simulink model "LKARefMdl"  (R2020b)
settings: Solver=FixedStepAuto  StartTime=0.0  StopTime=simStopTime  FixedStep=1e-3  RelTol=1e-3
values from neighbouring files (symbols this model uses):
  gammann = 10000    [CreateNnMatrices.m]    (also in HvsNN.m = 0.01; MPC_Constrained_Control.m; MPC_NN.m = 1e+15)
  nc = n_c    (= 8)    [Model_Init_Bayes.m]
  np = n_p    (= 24)    [Model_Init_Bayes.m]
  numbConstr = 3*nc + 2*np    [CreateNnMatrices.m]    (also in HvsNN.m; MPC_Constrained_Control.m; MPC_NN.m)
  PredictionHorizon = 30    [helperLKASetUp.m]
  Ts = 0.1    [Model_Init_Bayes.m]    (also in helperLKASetUp.m)
undefined symbols (not defined in the file or in its folder): DiscIntNeverNeededParam, K
libraries: simulink x13, pid_lib x2
(part 1 of 2)
settings Model: Creator=The MathWorks, Inc.  LastModifiedBy=Stage
settings DataIOCC: SaveOutput=off  SaveTime=off  ReturnWorkspaceOutputs=off
settings OptimizationCC: DefaultParameterBehavior=Inlined  UseFloatMulNetSlope=on  DefaultUnderspecifiedDataType=single  UseSpecifiedMinMax=on  InlineInvariantSignals=on  EnhancedBackFolding=on  StrengthReduction=on  PassReuseOutputArgsAs=Individual arguments  ZeroExternalMemoryAtStartup=off  ZeroInternalMemoryAtStartup=off  NoFixptDivByZeroProtection=on  EfficientFloat2IntCast=on  OptimizeBlockOrder=speed  DifferentSizesBufferReuse=on  EfficientTunableParamExpr=on
settings DebuggingCC: ParameterPrecisionLossMsg=none  ParameterTunabilityLossMsg=error  ArithmeticOperatorsInVariantConditions=warning
settings HardwareCC: ProdLongLongMode=on
settings ModelReferenceCC: ModelReferenceNumInstancesAllowed=Single
settings SFSimCC: SimUseLocalCustomCode=off  MATLABDynamicMemAlloc=off  CustomCodeUndefinedFunction=UseInterfaceOnly  SimTargetLang=C++
settings RTWCC: Description=Embedded Coder  SystemTargetFile=ert.tlc  TemplateMakefile=ert_default_tmf  GenerateReport=on  RTWUseLocalCustomCode=off  BuildConfiguration=Faster Runs  IncludeHyperlinkInReport=on  LaunchReport=on  TargetLang=C++  GenerateTraceInfo=on  GenerateTraceReport=on  GenerateTraceReportSl=on  GenerateTraceReportSf=on  GenerateTraceReportEml=on
settings CodeAppCC: ForceParamTrailComments=on  IgnoreCustomStorageClasses=off  OperatorAnnotations=on  SimulinkDataObjDesc=on  SFDataObjDesc=on  InsertBlockDesc=on
settings ERTTargetCC: TargetLangStandard=C++03 (ISO)  GenerateSampleERTMain=on  CombineSignalStateStructs=on  SuppressErrorStatus=on  CodeInterfacePackaging=C++ class  InlinedParameterPlacement=NonHierarchical  RootIOFormat=Structure reference  ERTCustomFileTemplate=example_file_process.tlc

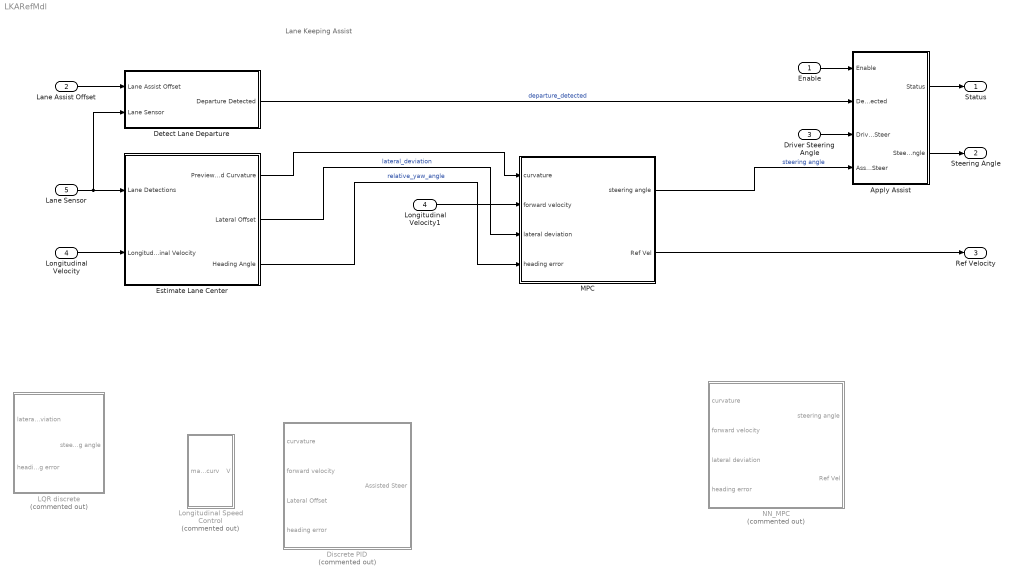
== system LKARefMdl ==
  note: Lane Keeping Assist
  Enable : Inport  OutDataTypeStr=boolean
  Lane Assist Offset : Inport  Port=2  OutDataTypeStr=single  Unit=m  SampleTime=Ts
  Driver Steering Angle : Inport  Port=3  Unit=rad
  Longitudinal Velocity : Inport  Port=4  OutDataTypeStr=single  Unit=m/s  SampleTime=Ts
  Lane Sensor : Inport  Port=5  OutDataTypeStr=Bus: LaneSensor  PortDimensions=[1 1]  SampleTime=Ts  BusOutputAsStruct=on
  Apply Assist : Subsystem
  Detect Lane Departure : Subsystem
  Discrete PID : Subsystem  Commented=on
  Estimate Lane Center : Subsystem  VariantControl=v2
  "LQR discrete " : Subsystem  Commented=on
  Longitudinal Speed Control : Subsystem  Commented=on
  Longitudinal Velocity1 : InportShadow  Port=4  OutDataTypeStr=single  Unit=m/s  SampleTime=Ts
  MPC : Subsystem
  NN_MPC : Subsystem  Commented=on
  Status : Outport  PortDimensions=1  VectorParamsAs1DForOutWhenUnconnected=off
  Steering Angle : Outport  Port=2  PortDimensions=1  VectorParamsAs1DForOutWhenUnconnected=off
  Ref Velocity : Outport  Port=3  PortDimensions=1  VectorParamsAs1DForOutWhenUnconnected=off
  wires:
  Estimate Lane Center/1(Previewed Curvature) -> MPC/1(curvature)
  Lane Assist Offset/1 -> Detect Lane Departure/1(Lane Assist Offset)
  Driver Steering Angle/1 -> Apply Assist/3(Driver Steer)
  Enable/1 -> Apply Assist/1(Enable)
  Apply Assist/1(Status) -> Status/1
  Apply Assist/2(Steering Angle) -> Steering Angle/1
  Detect Lane Departure/1(Departure Detected) -> Apply Assist/2(Departure Detected)  "departure_detected"
  Longitudinal Velocity/1 -> Estimate Lane Center/2(Longitudinal Velocity)
  Lane Sensor/1 -> Detect Lane Departure/2(Lane Sensor), Estimate Lane Center/1(Lane Detections)
  Estimate Lane Center/3(Heading Angle) -> MPC/4(heading error)  "relative_yaw_angle"
  Longitudinal Velocity1/1 -> MPC/2(forward velocity)
  MPC/2(Ref Vel) -> Ref Velocity/1
  MPC/1(steering angle) -> Apply Assist/4(Assisted Steer)  "steering angle"
  Estimate Lane Center/2(Lateral Offset) -> MPC/3(lateral deviation)  "lateral_deviation"

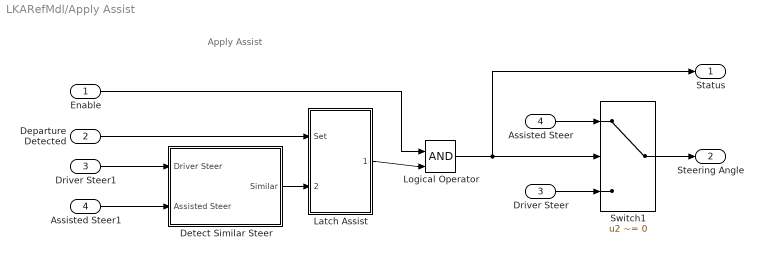
== system LKARefMdl/Apply Assist ==
  note: Apply Assist
  Enable : Inport
  Departure Detected : Inport  Port=2
  Driver Steer : Inport  Port=3
  Assisted Steer : Inport  Port=4
  Assisted Steer1 : InportShadow  Port=4
  "Detect Similar Steer " : Subsystem
  Driver Steer1 : InportShadow  Port=3
  Latch Assist : Subsystem
  Logical Operator : Logic  IconShape=distinctive  AllPortsSameDT=off  OutDataTypeStr=boolean
  Switch1 : Switch  Criteria=u2 ~= 0  Threshold=2
  Status : Outport  VectorParamsAs1DForOutWhenUnconnected=off
  Steering Angle : Outport  Port=2  Unit=rad  VectorParamsAs1DForOutWhenUnconnected=off
  wires:
  Assisted Steer/1 -> Switch1/1
  Driver Steer/1 -> Switch1/3
  Switch1/1 -> Steering Angle/1
  Enable/1 -> Logical Operator/1
  Logical Operator/1 -> Status/1, Switch1/2
  Driver Steer1/1 -> "Detect Similar Steer "/1(Driver Steer)
  Assisted Steer1/1 -> "Detect Similar Steer "/2(Assisted Steer)
  Departure Detected/1 -> Latch Assist/1(Set)
  "Detect Similar Steer "/1(Similar) -> Latch Assist/2(Reset)
  Latch Assist/1(Assist) -> Logical Operator/2

== system LKARefMdl/Detect Lane Departure ==
  note: Detect Lane Departure
  Lane Assist Offset : Inport
  In Bus Element : Inport  Port=2  PortName=Lane Sensor  Element=Left.LateralOffset
  In Bus Element1 : Inport  Port=2  PortName=Lane Sensor  Element=Right.LateralOffset
  Gain : Gain  Gain=-1
  Lane Assist Offset1 : InportShadow
  Logical Operator : Logic  Operator=OR  IconShape=distinctive  AllPortsSameDT=off  OutDataTypeStr=boolean
  Relational Operator : RelationalOperator  Operator=<=  OutDataTypeStr=boolean  RndMeth=Simplest
  Relational Operator1 : RelationalOperator  OutDataTypeStr=boolean  RndMeth=Simplest
  Departure Detected : Outport  VectorParamsAs1DForOutWhenUnconnected=off
  wires:
  Lane Assist Offset/1 -> Relational Operator/2  "left_assist_offset"
  In Bus Element/1 -> Relational Operator/1  "left_lateral_offset"
  Lane Assist Offset1/1 -> Gain/1  "left_assist_offset"
  In Bus Element1/1 -> Relational Operator1/1  "right_lateral_offset"
  Gain/1 -> Relational Operator1/2  "right_assist_offset"
  Relational Operator/1 -> Logical Operator/1
  Relational Operator1/1 -> Logical Operator/2
  Logical Operator/1 -> Departure Detected/1

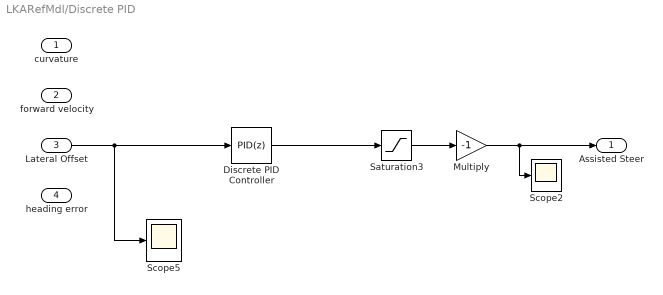
== system LKARefMdl/Discrete PID ==
  curvature : Inport
  forward velocity : Inport  Port=2
  Lateral Offset : Inport  Port=3
  heading error : Inport  Port=4
  Discrete PID Controller : pid_lib/PID Controller  Controller=PID  Form=Parallel  TimeDomain=Discrete-time  UseExternalTs=off  SampleTime=-1  IntegratorMethod=Forward Euler  FilterMethod=Forward Euler  ControllerParametersSource=internal  P=.5  I=.1  D=1  UseFilter=off  N=100  TunerSelectOption=Transfer Function Based (PID Tuner App)  InitialConditionSource=internal  InitialConditionForIntegrator=0  InitialConditionForFilter=0  DifferentiatorICPrevScaledInput=0  ExternalReset=none  TrackingMode=off  Kt=1  LimitOutput=off  SatLimitsSource=internal  UpperSaturationLimit=inf  LowerSaturationLimit=-inf  LinearizeAsGain=off  AntiWindupMode=none  Kb=1  POutMin=[]  POutMax=[]  IOutMin=[]  IOutMax=[]  DOutMin=[]  DOutMax=[]  NOutMin=[]  NOutMax=[]  SumOutMin=[]  SumOutMax=[]  SaturationOutMin=[]  SaturationOutMax=[]  PParamMin=[]  PParamMax=[]  IParamMin=[]  IParamMax=[]  DParamMin=[]  DParamMax=[]  NParamMin=[]  NParamMax=[]  KbParamMin=[]  KbParamMax=[]  KtParamMin=[]  KtParamMax=[]  KbOutMin=[]  KbOutMax=[]  KtOutMin=[]  KtOutMax=[]  IntegratorOutMin=[]  IntegratorOutMax=[]  FilterOutMin=[]  FilterOutMax=[]  SumI1OutMin=[]  SumI1OutMax=[]  SumI2OutMin=[]  SumI2OutMax=[]  SumI3OutMin=[]  SumI3OutMax=[]  SumI4OutMin=[]  SumI4OutMax=[]  SumDOutMin=[]  SumDOutMax=[]  DifferentiatorOutMin=[]  DifferentiatorOutMax=[]  FilterDiffOutCoefMin=[]  FilterDiffOutCoefMax=[]  ReciprocalOutMin=[]  ReciprocalOutMax=[]  SumDenOutMin=[]  SumDenOutMax=[]  SumNumOutMin=[]  SumNumOutMax=[]  DivideOutMin=[]  DivideOutMax=[]  UdiffTsProdOutMin=[]  UdiffTsProdOutMax=[]  NTsProdOutMin=[]  NTsProdOutMax=[]  UintegralTsProdOutMin=[]  UintegralTsProdOutMax=[]  UngainTsProdOutMin=[]  UngainTsProdOutMax=[]  IntegratorContinuousStateAttributes=''  IntegratorStateMustResolveToSignalObject=off  IntegratorRTWStateStorageClass=Auto  FilterContinuousStateAttributes=''  FilterStateMustResolveToSignalObject=off  FilterRTWStateStorageClass=Auto  ParallelPVariant=InternalParameters  IdealPVariant=Disabled  IVariant=InternalParameters  DVariant=InternalParameters  IntegratorVariant=Discrete  SatVariant=Disabled  AWVariant=Passthrough  PCopyVariant=Disabled  TRVariant=Disabled  FdbkBlocksVariant=Forward  IdealPFdbkVariant=Disabled  SatFdbkVariant=Disabled  DerivativeFilterVariant=Differentiator  NVariant=Passthrough  NCopyVariant=Disabled_SignalSpec  FilterICVariant=InternalICsDifferentiator  IntegratorICVariant=InternalICs  ExternalResetVariant=Disabled  TRSumVariant=Passthrough  SumFdbkVariant=Disabled  SumVariant=Sum_PID  TsampFilterVariant=InternalTs  TsampNgainVariant=Passthrough  TsampIntegralVariant=Passthrough  ExternalSaturationOutDataTypeStr=Inherit: Same as second input
  Multiply : Gain  Gain=-1
  Saturation3 : Saturate
  Scope2 : Scope
  Scope5 : Scope
  Assisted Steer : Outport
  wires:
  Lateral Offset/1 -> Discrete PID Controller/1, Scope5/1
  Discrete PID Controller/1 -> Saturation3/1
  Saturation3/1 -> Multiply/1
  Multiply/1 -> Scope2/1, Assisted Steer/1

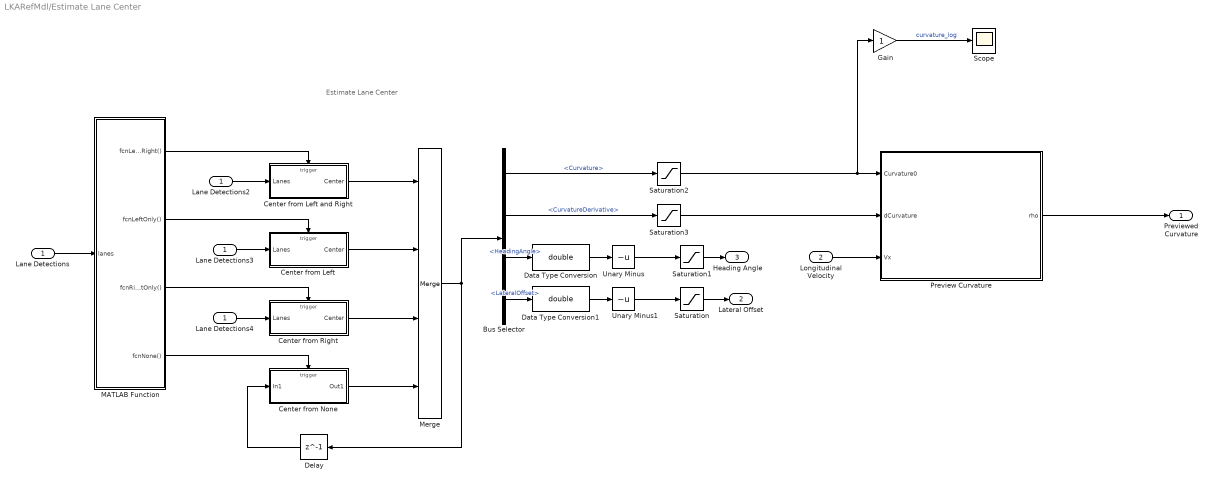
== system LKARefMdl/Estimate Lane Center ==
  note: Estimate Lane Center
  Lane Detections : Inport
  Longitudinal Velocity : Inport  Port=2  OutDataTypeStr=single
  Bus Selector : BusSelector  OutputSignals=Curvature,CurvatureDerivative,HeadingAngle,LateralOffset
  Center from Left : Subsystem  TreatAsAtomicUnit=on
  Center from Left and Right : Subsystem  TreatAsAtomicUnit=on
  Center from None : Subsystem  TreatAsAtomicUnit=on
  Center from Right : Subsystem  TreatAsAtomicUnit=on
  Data Type Conversion : DataTypeConversion  OutDataTypeStr=double
  Data Type Conversion1 : DataTypeConversion  OutDataTypeStr=double
  Delay : Delay  DelayLength=1
  Gain : Gain
  Lane Detections2 : InportShadow
  Lane Detections3 : InportShadow
  Lane Detections4 : InportShadow
  MATLAB Function : MATLAB Function  TreatAsAtomicUnit=on
  Merge : Merge  Inputs=4
  Preview Curvature : MATLAB Function  TreatAsAtomicUnit=on  SystemSampleTime=Ts
  Saturation : Saturate
  Saturation1 : Saturate  UpperLimit=0.6  LowerLimit=-0.6
  Saturation2 : Saturate  UpperLimit=0.15  LowerLimit=-0.15
  Saturation3 : Saturate  UpperLimit=0.06  LowerLimit=-0.06
  Scope : Scope
  Unary Minus : UnaryMinus
  Unary Minus1 : UnaryMinus
  Previewed Curvature : Outport  VectorParamsAs1DForOutWhenUnconnected=off
  Lateral Offset : Outport  Port=2  VectorParamsAs1DForOutWhenUnconnected=off
  Heading Angle : Outport  Port=3  VectorParamsAs1DForOutWhenUnconnected=off
  wires:
  Bus Selector/3 -> Data Type Conversion/1  "<HeadingAngle>"
  Bus Selector/4 -> Data Type Conversion1/1  "<LateralOffset>"
  Unary Minus1/1 -> Saturation/1
  Bus Selector/1 -> Saturation2/1  "<Curvature>"
  Bus Selector/2 -> Saturation3/1  "<CurvatureDerivative>"
  Longitudinal Velocity/1 -> Preview Curvature/3(Vx)
  Unary Minus/1 -> Saturation1/1
  Saturation/1 -> Lateral Offset/1
  Saturation1/1 -> Heading Angle/1
  Saturation3/1 -> Preview Curvature/2(dCurvature)
  Merge/1 -> Delay/1, Bus Selector/1
  Center from Left/1(Center) -> Merge/2
  MATLAB Function/4(fcnNone()) -> Center from None/Trigger
  MATLAB Function/3(fcnRightOnly()) -> Center from Right/Trigger
  Lane Detections2/1 -> Center from Left and Right/1(Lanes)
  Lane Detections/1 -> MATLAB Function/1(lanes)
  Center from Left and Right/1(Center) -> Merge/1
  Delay/1 -> Center from None/1(In1)
  MATLAB Function/1(fcnLeftAndRight()) -> Center from Left and Right/Trigger
  Center from None/1(Out1) -> Merge/4
  MATLAB Function/2(fcnLeftOnly()) -> Center from Left/Trigger
  Lane Detections4/1 -> Center from Right/1(Lanes)
  Lane Detections3/1 -> Center from Left/1(Lanes)
  Center from Right/1(Center) -> Merge/3
  Data Type Conversion/1 -> Unary Minus/1
  Data Type Conversion1/1 -> Unary Minus1/1
  Preview Curvature/1(rho) -> Previewed Curvature/1
  Gain/1 -> Scope/1  "curvature_log"
  Saturation2/1 -> Gain/1, Preview Curvature/1(Curvature0)

== system LKARefMdl/LQR discrete  ==
  lateral deviation : Inport
  heading error : Inport  Port=2
  Discrete Derivative : simulink/Discrete/Discrete Derivative  gainval=1.0  ICPrevScaledInput=0.0  OutMin=[]  OutMax=[]  OutDataType=fixdt(1, 16)  OutScaling=2^-10  DoSatur=off
  Discrete Derivative1 : simulink/Discrete/Discrete Derivative  gainval=1.0  ICPrevScaledInput=0.012353340233836  OutMin=[]  OutMax=[]  OutDataType=fixdt(1, 16)  OutScaling=2^-10  DoSatur=off
  Multiply : Gain  Gain=-K  Multiplication=Matrix(K*u) (u vector)
  Mux : Mux
  Saturation : Saturate  UpperLimit=0.4  LowerLimit=-0.4
  steering angle : Outport
  wires:
  Multiply/1 -> Saturation/1
  Saturation/1 -> steering angle/1
  Discrete Derivative1/1 -> Mux/4
  Discrete Derivative/1 -> Mux/2
  Mux/1 -> Multiply/1
  lateral deviation/1 -> Discrete Derivative/1, Mux/1
  heading error/1 -> Mux/3, Discrete Derivative1/1

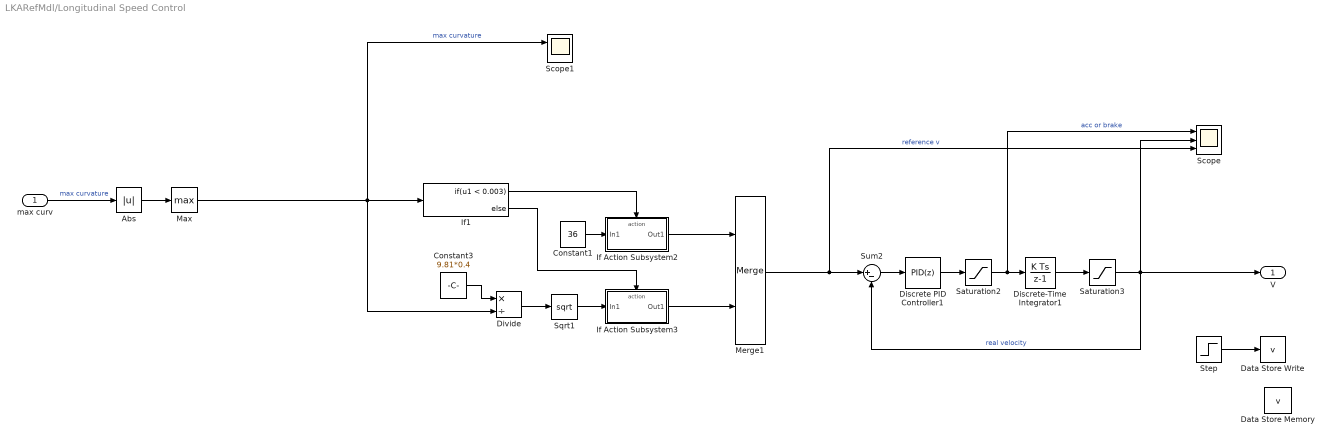
== system LKARefMdl/Longitudinal Speed Control ==
  max curv : Inport
  Abs : Abs
  Constant1 : Constant  Value=36
  Constant3 : Constant  Value=9.81*0.4
  Data Store Memory : DataStoreMemory  DataStoreName=v  ReadBeforeWriteMsg=warning  WriteAfterWriteMsg=warning  WriteAfterReadMsg=warning  ShowAdditionalParam=off  OutDataTypeStr=double
  Data Store Write : DataStoreWrite  DataStoreName=v  DataStoreElements=v
  Discrete PID Controller1 : pid_lib/PID Controller  Controller=PID  Form=Parallel  TimeDomain=Discrete-time  UseExternalTs=off  SampleTime=Ts  IntegratorMethod=Forward Euler  FilterMethod=Forward Euler  ControllerParametersSource=internal  P=7  I=0  D=0  UseFilter=on  N=100  TunerSelectOption=Transfer Function Based (PID Tuner App)  InitialConditionSource=internal  InitialConditionForIntegrator=0  InitialConditionForFilter=0  DifferentiatorICPrevScaledInput=0  ExternalReset=none  TrackingMode=off  Kt=1  LimitOutput=off  SatLimitsSource=internal  UpperSaturationLimit=inf  LowerSaturationLimit=-inf  LinearizeAsGain=off  AntiWindupMode=none  Kb=1  POutMin=[]  POutMax=[]  IOutMin=[]  IOutMax=[]  DOutMin=[]  DOutMax=[]  NOutMin=[]  NOutMax=[]  SumOutMin=[]  SumOutMax=[]  SaturationOutMin=[]  SaturationOutMax=[]  PParamMin=[]  PParamMax=[]  IParamMin=[]  IParamMax=[]  DParamMin=[]  DParamMax=[]  NParamMin=[]  NParamMax=[]  KbParamMin=[]  KbParamMax=[]  KtParamMin=[]  KtParamMax=[]  KbOutMin=[]  KbOutMax=[]  KtOutMin=[]  KtOutMax=[]  IntegratorOutMin=[]  IntegratorOutMax=[]  FilterOutMin=[]  FilterOutMax=[]  SumI1OutMin=[]  SumI1OutMax=[]  SumI2OutMin=[]  SumI2OutMax=[]  SumI3OutMin=[]  SumI3OutMax=[]  SumI4OutMin=[]  SumI4OutMax=[]  SumDOutMin=[]  SumDOutMax=[]  DifferentiatorOutMin=[]  DifferentiatorOutMax=[]  FilterDiffOutCoefMin=[]  FilterDiffOutCoefMax=[]  ReciprocalOutMin=[]  ReciprocalOutMax=[]  SumDenOutMin=[]  SumDenOutMax=[]  SumNumOutMin=[]  SumNumOutMax=[]  DivideOutMin=[]  DivideOutMax=[]  UdiffTsProdOutMin=[]  UdiffTsProdOutMax=[]  NTsProdOutMin=[]  NTsProdOutMax=[]  UintegralTsProdOutMin=[]  UintegralTsProdOutMax=[]  UngainTsProdOutMin=[]  UngainTsProdOutMax=[]  IntegratorContinuousStateAttributes=''  IntegratorStateMustResolveToSignalObject=off  IntegratorRTWStateStorageClass=Auto  FilterContinuousStateAttributes=''  FilterStateMustResolveToSignalObject=off  FilterRTWStateStorageClass=Auto  ParallelPVariant=InternalParameters  IdealPVariant=Disabled  IVariant=InternalParameters  DVariant=InternalParameters  IntegratorVariant=Discrete  SatVariant=Disabled  AWVariant=Passthrough  PCopyVariant=Disabled  TRVariant=Disabled  FdbkBlocksVariant=Forward  IdealPFdbkVariant=Disabled  SatFdbkVariant=Disabled  DerivativeFilterVariant=ForwardEulerFilter  NVariant=InternalParameters  NCopyVariant=Disabled  FilterICVariant=InternalICsFilter  IntegratorICVariant=InternalICs  ExternalResetVariant=Disabled  TRSumVariant=Passthrough  SumFdbkVariant=Disabled  SumVariant=Sum_PID  TsampFilterVariant=InternalTs  TsampNgainVariant=Passthrough  TsampIntegralVariant=Passthrough  ExternalSaturationOutDataTypeStr=Inherit: Same as second input
  Discrete-Time Integrator1 : DiscreteIntegrator  SampleTime=Ts  ICPrevOutput=DiscIntNeverNeededParam  ICPrevScaledInput=DiscIntNeverNeededParam
  Divide : Product  Inputs=*/
  If Action Subsystem2 : Subsystem  TreatAsAtomicUnit=on
  If Action Subsystem3 : Subsystem  TreatAsAtomicUnit=on
  If1 : If  IfExpression=u1 < 0.003
  Max : MinMax  Function=max
  Merge1 : Merge
  Saturation2 : Saturate  UpperLimit=0.5*9.81  LowerLimit=-0.5*9.81
  Saturation3 : Saturate  UpperLimit=36  LowerLimit=0
  Scope : Scope  NumInputPorts=3
  Scope1 : Scope  NumInputPorts=2
  Sqrt1 : Sqrt  SaturateOnIntegerOverflow=on
  Step : Step  Time=5  Before=2  After=7  SampleTime=0
  Sum2 : Sum  Inputs=|+-
  V : Outport
  wires:
  Saturation3/1 -> V/1, Sum2/2, Scope/2  "real velocity"
  Saturation2/1 -> Scope/1, Discrete-Time Integrator1/1  "acc or brake"
  Discrete-Time Integrator1/1 -> Saturation3/1
  Discrete PID Controller1/1 -> Saturation2/1
  Sum2/1 -> Discrete PID Controller1/1
  Merge1/1 -> Scope/3, Sum2/1  "reference v"
  If1/1 -> If Action Subsystem2/Action
  Constant3/1 -> Divide/1
  Max/1 -> Divide/2, Scope1/1, If1/1  "max curvature"
  Constant1/1 -> If Action Subsystem2/1(In1)
  If Action Subsystem2/1(Out1) -> Merge1/1
  Divide/1 -> Sqrt1/1
  Sqrt1/1 -> If Action Subsystem3/1(In1)
  If1/2 -> If Action Subsystem3/Action
  If Action Subsystem3/1(Out1) -> Merge1/2
  Step/1 -> Data Store Write/1
  Abs/1 -> Max/1
  max curv/1 -> Abs/1  "max curvature"

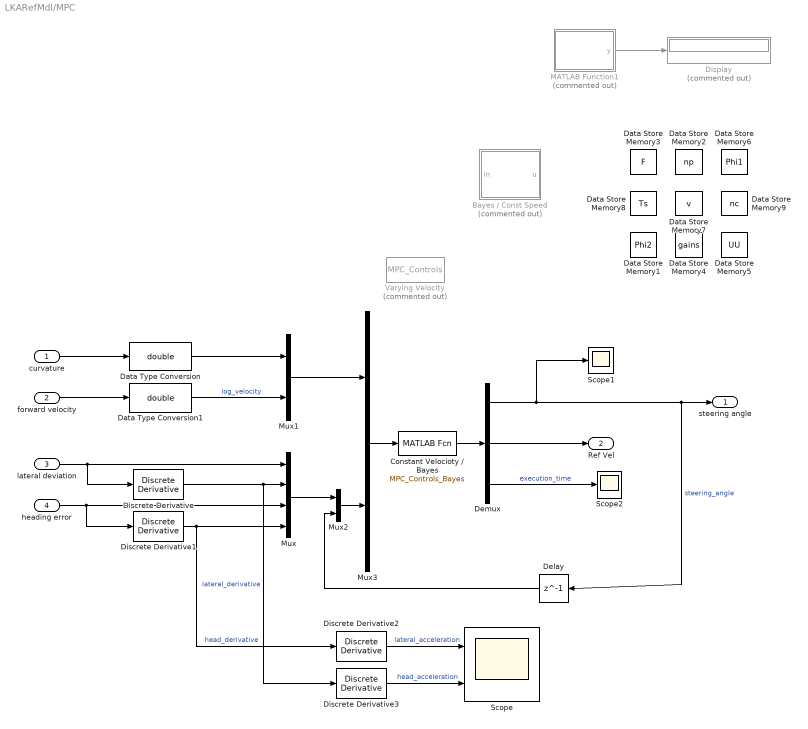
== system LKARefMdl/MPC ==
  curvature : Inport
  forward velocity : Inport  Port=2
  lateral deviation : Inport  Port=3
  heading error : Inport  Port=4
  Bayes / Const Speed : MATLAB Function  Commented=on  TreatAsAtomicUnit=on
  Constant Velocioty / Bayes : MATLABFcn  MATLABFcn=MPC_Controls_Bayes  OutputDimensions=3  OutputSignalType=real  Output1D=off
  Data Store Memory1 : DataStoreMemory  DataStoreName=Phi2  WriteAfterWriteMsg=warning  WriteAfterReadMsg=warning  InitialValue=Phi2  ShowAdditionalParam=off  OutDataTypeStr=double
  Data Store Memory2 : DataStoreMemory  DataStoreName=np  WriteAfterWriteMsg=warning  WriteAfterReadMsg=warning  InitialValue=np  ShowAdditionalParam=off  OutDataTypeStr=double
  Data Store Memory3 : DataStoreMemory  DataStoreName=F  WriteAfterWriteMsg=warning  WriteAfterReadMsg=warning  InitialValue=F  ShowAdditionalParam=off  OutDataTypeStr=double
  Data Store Memory4 : DataStoreMemory  DataStoreName=gains  WriteAfterWriteMsg=warning  WriteAfterReadMsg=warning  InitialValue=gains  ShowAdditionalParam=off  OutDataTypeStr=double
  Data Store Memory5 : DataStoreMemory  DataStoreName=UU  WriteAfterWriteMsg=warning  WriteAfterReadMsg=warning  InitialValue=UU  ShowAdditionalParam=off  OutDataTypeStr=double
  Data Store Memory6 : DataStoreMemory  DataStoreName=Phi1  WriteAfterWriteMsg=warning  WriteAfterReadMsg=warning  InitialValue=Phi2  ShowAdditionalParam=off  OutDataTypeStr=double
  Data Store Memory7 : DataStoreMemory  DataStoreName=v  WriteAfterWriteMsg=warning  WriteAfterReadMsg=warning  InitialValue=v  ShowAdditionalParam=off  OutDataTypeStr=double
  Data Store Memory8 : DataStoreMemory  DataStoreName=Ts  WriteAfterWriteMsg=warning  WriteAfterReadMsg=warning  InitialValue=Ts  ShowAdditionalParam=off  OutDataTypeStr=double
  Data Store Memory9 : DataStoreMemory  DataStoreName=nc  WriteAfterWriteMsg=warning  WriteAfterReadMsg=warning  InitialValue=nc  ShowAdditionalParam=off  OutDataTypeStr=double
  Data Type Conversion : DataTypeConversion  OutDataTypeStr=double
  Data Type Conversion1 : DataTypeConversion  OutDataTypeStr=double
  Delay : Delay  DelayLength=1  InitialCondition=0
  Demux : Demux  Outputs=3
  Discrete Derivative : simulink/Discrete/Discrete Derivative  gainval=1.0  ICPrevScaledInput=10  OutMin=[]  OutMax=[]  OutDataType=fixdt(1, 16)  OutScaling=2^-10  DoSatur=off
  Discrete Derivative1 : simulink/Discrete/Discrete Derivative  gainval=1.0  ICPrevScaledInput=0.0  OutMin=[]  OutMax=[]  OutDataType=fixdt(1, 16)  OutScaling=2^-10  DoSatur=off
  Discrete Derivative2 : simulink/Discrete/Discrete Derivative  gainval=1.0  ICPrevScaledInput=10  OutMin=[]  OutMax=[]  OutDataType=fixdt(1, 16)  OutScaling=2^-10  DoSatur=off
  Discrete Derivative3 : simulink/Discrete/Discrete Derivative  gainval=1.0  ICPrevScaledInput=0.0  OutMin=[]  OutMax=[]  OutDataType=fixdt(1, 16)  OutScaling=2^-10  DoSatur=off
  Display : Display  Commented=on
  MATLAB Function1 : MATLAB Function  Commented=on  TreatAsAtomicUnit=on
  Mux : Mux
  Mux1 : Mux  Inputs=2
  Mux2 : Mux  Inputs=2
  Mux3 : Mux  Inputs=2
  Scope : Scope  NumInputPorts=2
  Scope1 : Scope
  Scope2 : Scope
  Varying Velocity : MATLABFcn  Commented=on  MATLABFcn=MPC_Controls  OutputDimensions=2  OutputSignalType=real  Output1D=off
  steering angle : Outport
  Ref Vel : Outport  Port=2
  wires:
  Constant Velocioty / Bayes/1 -> Demux/1
  Mux3/1 -> Constant Velocioty / Bayes/1
  Discrete Derivative2/1 -> Scope/1  "lateral_acceleration"
  Discrete Derivative3/1 -> Scope/2  "head_acceleration"
  Delay/1 -> Mux2/2
  Demux/2 -> Ref Vel/1
  Data Type Conversion1/1 -> Mux1/2  "log_velocity"
  MATLAB Function1/1(y) -> Display/1
  Mux1/1 -> Mux3/1
  Mux2/1 -> Mux3/2
  Mux/1 -> Mux2/1
  Data Type Conversion/1 -> Mux1/1
  forward velocity/1 -> Data Type Conversion1/1
  Demux/1 -> Delay/1, steering angle/1, Scope1/1  "steering_angle"
  Discrete Derivative/1 -> Discrete Derivative3/1, Mux/2  "lateral_derivative"
  Discrete Derivative1/1 -> Mux/4, Discrete Derivative2/1  "head_derivative"
  heading error/1 -> Mux/3, Discrete Derivative1/1
  lateral deviation/1 -> Discrete Derivative/1, Mux/1
  curvature/1 -> Data Type Conversion/1
  Demux/3 -> Scope2/1  "execution_time"

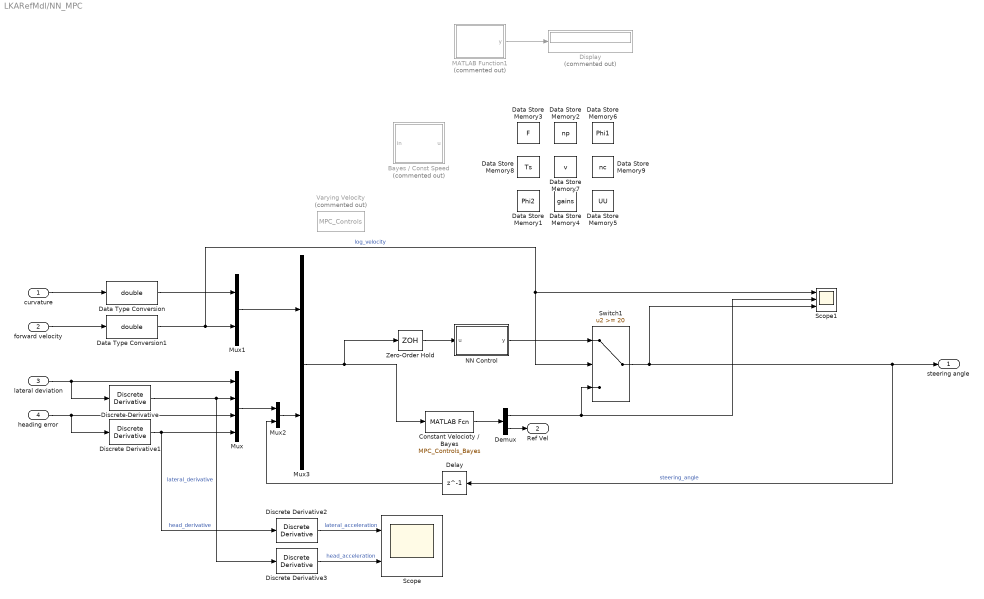
== system LKARefMdl/NN_MPC ==
  curvature : Inport
  forward velocity : Inport  Port=2
  lateral deviation : Inport  Port=3
  heading error : Inport  Port=4
  Bayes / Const Speed : MATLAB Function  Commented=on  TreatAsAtomicUnit=on
  Constant Velocioty / Bayes : MATLABFcn  MATLABFcn=MPC_Controls_Bayes  OutputDimensions=2  OutputSignalType=real  Output1D=off
  Data Store Memory1 : DataStoreMemory  DataStoreName=Phi2  WriteAfterWriteMsg=warning  WriteAfterReadMsg=warning  InitialValue=Phi2  ShowAdditionalParam=off  OutDataTypeStr=double
  Data Store Memory2 : DataStoreMemory  DataStoreName=np  WriteAfterWriteMsg=warning  WriteAfterReadMsg=warning  InitialValue=np  ShowAdditionalParam=off  OutDataTypeStr=double
  Data Store Memory3 : DataStoreMemory  DataStoreName=F  WriteAfterWriteMsg=warning  WriteAfterReadMsg=warning  InitialValue=F  ShowAdditionalParam=off  OutDataTypeStr=double
  Data Store Memory4 : DataStoreMemory  DataStoreName=gains  WriteAfterWriteMsg=warning  WriteAfterReadMsg=warning  InitialValue=gains  ShowAdditionalParam=off  OutDataTypeStr=double
  Data Store Memory5 : DataStoreMemory  DataStoreName=UU  WriteAfterWriteMsg=warning  WriteAfterReadMsg=warning  InitialValue=UU  ShowAdditionalParam=off  OutDataTypeStr=double
  Data Store Memory6 : DataStoreMemory  DataStoreName=Phi1  WriteAfterWriteMsg=warning  WriteAfterReadMsg=warning  InitialValue=Phi1  ShowAdditionalParam=off  OutDataTypeStr=double
  Data Store Memory7 : DataStoreMemory  DataStoreName=v  WriteAfterWriteMsg=warning  WriteAfterReadMsg=warning  InitialValue=v  ShowAdditionalParam=off  OutDataTypeStr=double
  Data Store Memory8 : DataStoreMemory  DataStoreName=Ts  WriteAfterWriteMsg=warning  WriteAfterReadMsg=warning  InitialValue=Ts  ShowAdditionalParam=off  OutDataTypeStr=double
  Data Store Memory9 : DataStoreMemory  DataStoreName=nc  WriteAfterWriteMsg=warning  WriteAfterReadMsg=warning  InitialValue=nc  ShowAdditionalParam=off  OutDataTypeStr=double
  Data Type Conversion : DataTypeConversion  OutDataTypeStr=double
  Data Type Conversion1 : DataTypeConversion  OutDataTypeStr=double
  Delay : Delay  DelayLength=1  InitialCondition=0  SampleTime=Ts
  Demux : Demux  Outputs=2
  Discrete Derivative : simulink/Discrete/Discrete Derivative  gainval=1.0  ICPrevScaledInput=10  OutMin=[]  OutMax=[]  OutDataType=fixdt(1, 16)  OutScaling=2^-10  DoSatur=off
  Discrete Derivative1 : simulink/Discrete/Discrete Derivative  gainval=1.0  ICPrevScaledInput=0.0  OutMin=[]  OutMax=[]  OutDataType=fixdt(1, 16)  OutScaling=2^-10  DoSatur=off
  Discrete Derivative2 : simulink/Discrete/Discrete Derivative  gainval=1.0  ICPrevScaledInput=10  OutMin=[]  OutMax=[]  OutDataType=fixdt(1, 16)  OutScaling=2^-10  DoSatur=off
  Discrete Derivative3 : simulink/Discrete/Discrete Derivative  gainval=1.0  ICPrevScaledInput=0.0  OutMin=[]  OutMax=[]  OutDataType=fixdt(1, 16)  OutScaling=2^-10  DoSatur=off
  Display : Display  Commented=on
  MATLAB Function1 : MATLAB Function  Commented=on  TreatAsAtomicUnit=on
  Mux : Mux
  Mux1 : Mux  Inputs=2
  Mux2 : Mux  Inputs=2
  Mux3 : Mux  Inputs=2
  NN Control : Subsystem  TreatAsAtomicUnit=on
  Scope : Scope  NumInputPorts=2
  Scope1 : Scope  NumInputPorts=3
  Switch1 : Switch  Threshold=20
  Varying Velocity : MATLABFcn  Commented=on  MATLABFcn=MPC_Controls  OutputDimensions=2  OutputSignalType=real  Output1D=off
  Zero-Order Hold : ZeroOrderHold  SampleTime=0.00000001
  steering angle : Outport
  Ref Vel : Outport  Port=2
  wires:
  curvature/1 -> Data Type Conversion/1
  lateral deviation/1 -> Mux/1, Discrete Derivative/1
  heading error/1 -> Discrete Derivative1/1, Mux/3
  Discrete Derivative1/1 -> Discrete Derivative2/1, Mux/4  "head_derivative"
  Discrete Derivative/1 -> Mux/2, Discrete Derivative3/1  "lateral_derivative"
  Switch1/1 -> Scope1/3, steering angle/1, Delay/1  "steering_angle"
  forward velocity/1 -> Data Type Conversion1/1
  Data Type Conversion/1 -> Mux1/1
  Mux/1 -> Mux2/1
  Mux2/1 -> Mux3/2
  Mux1/1 -> Mux3/1
  MATLAB Function1/1(y) -> Display/1
  Data Type Conversion1/1 -> Scope1/1, Switch1/2, Mux1/2  "log_velocity"
  Delay/1 -> Mux2/2
  Discrete Derivative3/1 -> Scope/2  "head_acceleration"
  Discrete Derivative2/1 -> Scope/1  "lateral_acceleration"
  Mux3/1 -> Constant Velocioty / Bayes/1, Zero-Order Hold/1
  Demux/2 -> Ref Vel/1
  Constant Velocioty / Bayes/1 -> Demux/1
  Demux/1 -> Scope1/2, Switch1/3
  NN Control/1(y) -> Switch1/1
  Zero-Order Hold/1 -> NN Control/1(u)

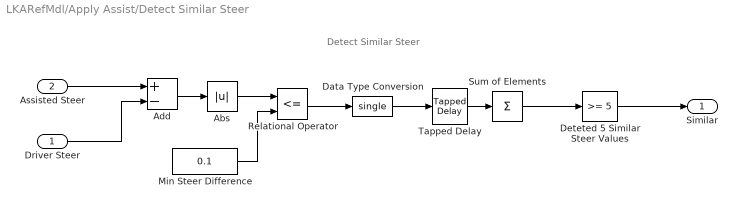
== system LKARefMdl/Apply Assist/Detect Similar Steer  ==
  note: Detect Similar Steer
  Driver Steer : Inport
  Assisted Steer : Inport  Port=2
  Abs : Abs
  Add : Sum  Inputs=+-
  Data Type Conversion : DataTypeConversion  OutDataTypeStr=single
  Deteted 5 Similar Steer Values : simulink/Logic and Bit Operations/Compare To Constant  relop=>=  const=5  OutDataTypeStr=boolean
  Min Steer Difference : Constant  Value=0.1
  Relational Operator : RelationalOperator  Operator=<=  OutDataTypeStr=boolean  RndMeth=Simplest
  Sum of Elements : Sum  Inputs=+
  Tapped Delay : simulink/Discrete/Tapped Delay  vinit=0.0  samptime=-1  NumDelays=5  DelayOrder=Oldest  includeCurrent=off
  Similar : Outport  VectorParamsAs1DForOutWhenUnconnected=off
  wires:
  Assisted Steer/1 -> Add/1
  Driver Steer/1 -> Add/2
  Add/1 -> Abs/1
  Relational Operator/1 -> Data Type Conversion/1
  Abs/1 -> Relational Operator/1
  Deteted 5 Similar Steer Values/1 -> Similar/1
  Min Steer Difference/1 -> Relational Operator/2
  Data Type Conversion/1 -> Tapped Delay/1
  Tapped Delay/1 -> Sum of Elements/1
  Sum of Elements/1 -> Deteted 5 Similar Steer Values/1

== system LKARefMdl/Apply Assist/Latch Assist ==
  note: Latch Assist
  Set : Inport
  Reset : Inport  Port=2
  Delay : Delay  DelayLength=1
  Logical Operator1 : Logic  Operator=OR  IconShape=distinctive  AllPortsSameDT=off  OutDataTypeStr=boolean
  Logical Operator2 : Logic  IconShape=distinctive  AllPortsSameDT=off  OutDataTypeStr=boolean
  Logical Operator3 : Logic  Operator=NOT  IconShape=distinctive  AllPortsSameDT=off  OutDataTypeStr=boolean
  Assist : Outport  VectorParamsAs1DForOutWhenUnconnected=off
  wires:
  Logical Operator1/1 -> Assist/1, Delay/1  "latch_assist"
  Delay/1 -> Logical Operator2/2
  Reset/1 -> Logical Operator3/1
  Logical Operator2/1 -> Logical Operator1/2  "unlatch_assist"
  Set/1 -> Logical Operator1/1
  Logical Operator3/1 -> Logical Operator2/1

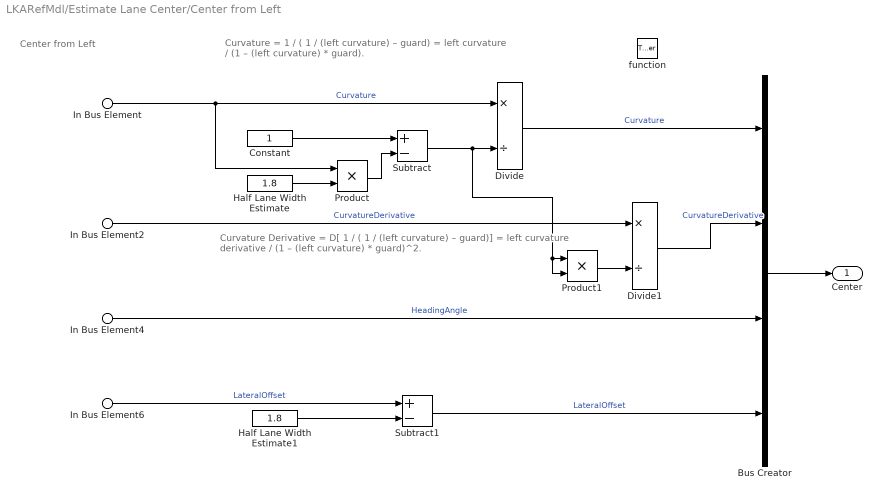
== system LKARefMdl/Estimate Lane Center/Center from Left ==
  note: Curvature
      | = 1 / ( 1 / (left curvature) – guard)
      | = left curvature / (1 – (left curvature) * guard).
  note: Center from Left
  note: Curvature Derivative
      | = D[ 1 / ( 1 / (left curvature) – guard)]
      | = left curvature derivative / (1 – (left curvature) * guard)^2.
  In Bus Element : Inport  PortName=Lanes  Element=Left.Curvature
  In Bus Element2 : Inport  PortName=Lanes  Element=Left.CurvatureDerivative
  In Bus Element4 : Inport  PortName=Lanes  Element=Left.HeadingAngle
  In Bus Element6 : Inport  PortName=Lanes  Element=Left.LateralOffset
  function : TriggerPort  TriggerType=function-call  VariantControl=Variant
  Bus Creator : BusCreator  Inputs=4
  Constant : Constant  OutDataTypeStr=Inherit: Inherit via back propagation
  Divide : Product  Inputs=*/
  Divide1 : Product  Inputs=*/
  Half Lane Width Estimate : Constant  Value=1.8  OutDataTypeStr=Inherit: Inherit via back propagation
  Half Lane Width Estimate1 : Constant  Value=1.8  OutDataTypeStr=Inherit: Inherit via back propagation
  Product : Product
  Product1 : Product
  Subtract : Sum  Inputs=+-
  Subtract1 : Sum  Inputs=+-
  Center : Outport  VectorParamsAs1DForOutWhenUnconnected=off
  wires:
  Bus Creator/1 -> Center/1
  Divide1/1 -> Bus Creator/2  "CurvatureDerivative"
  Divide/1 -> Bus Creator/1  "Curvature"
  In Bus Element4/1 -> Bus Creator/3  "HeadingAngle"
  Subtract1/1 -> Bus Creator/4  "LateralOffset"
  In Bus Element/1 -> Product/1, Divide/1  "Curvature"
  Subtract/1 -> Product1/2, Product1/1, Divide/2
  Half Lane Width Estimate/1 -> Product/2
  Constant/1 -> Subtract/1
  In Bus Element2/1 -> Divide1/1  "CurvatureDerivative"
  Product1/1 -> Divide1/2
  In Bus Element6/1 -> Subtract1/1  "LateralOffset"
  Half Lane Width Estimate1/1 -> Subtract1/2
  Product/1 -> Subtract/2

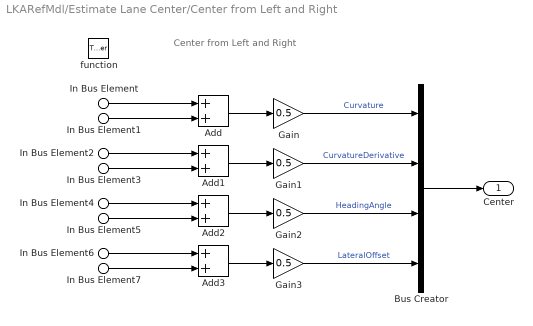
== system LKARefMdl/Estimate Lane Center/Center from Left and Right ==
  note: Center from Left and Right
  In Bus Element : Inport  PortName=Lanes  Element=Left.Curvature
  In Bus Element2 : Inport  PortName=Lanes  Element=Left.CurvatureDerivative
  In Bus Element4 : Inport  PortName=Lanes  Element=Left.HeadingAngle
  In Bus Element6 : Inport  PortName=Lanes  Element=Left.LateralOffset
  In Bus Element1 : Inport  PortName=Lanes  Element=Right.Curvature
  In Bus Element3 : Inport  PortName=Lanes  Element=Right.CurvatureDerivative
  In Bus Element5 : Inport  PortName=Lanes  Element=Right.HeadingAngle
  In Bus Element7 : Inport  PortName=Lanes  Element=Right.LateralOffset
  function : TriggerPort  TriggerType=function-call  VariantControl=Variant
  Add{,1..3} (4 alike) : Sum
  Bus Creator : BusCreator  Inputs=4
  Gain{,1..3} (4 alike) : Gain  Gain=0.5
  Center : Outport  VectorParamsAs1DForOutWhenUnconnected=off
  wires:
  Add/1 -> Gain/1
  Gain/1 -> Bus Creator/1  "Curvature"
  Add1/1 -> Gain1/1
  Gain1/1 -> Bus Creator/2  "CurvatureDerivative"
  Add2/1 -> Gain2/1
  Gain2/1 -> Bus Creator/3  "HeadingAngle"
  Add3/1 -> Gain3/1
  Gain3/1 -> Bus Creator/4  "LateralOffset"
  Bus Creator/1 -> Center/1
  In Bus Element/1 -> Add/1
  In Bus Element1/1 -> Add/2
  In Bus Element2/1 -> Add1/1
  In Bus Element3/1 -> Add1/2
  In Bus Element4/1 -> Add2/1
  In Bus Element5/1 -> Add2/2
  In Bus Element7/1 -> Add3/2
  In Bus Element6/1 -> Add3/1

== system LKARefMdl/Estimate Lane Center/Center from None ==
  In1 : Inport
  function : TriggerPort  TriggerType=function-call  VariantControl=Variant
  Out1 : Outport  VectorParamsAs1DForOutWhenUnconnected=off
  wires:
  In1/1 -> Out1/1

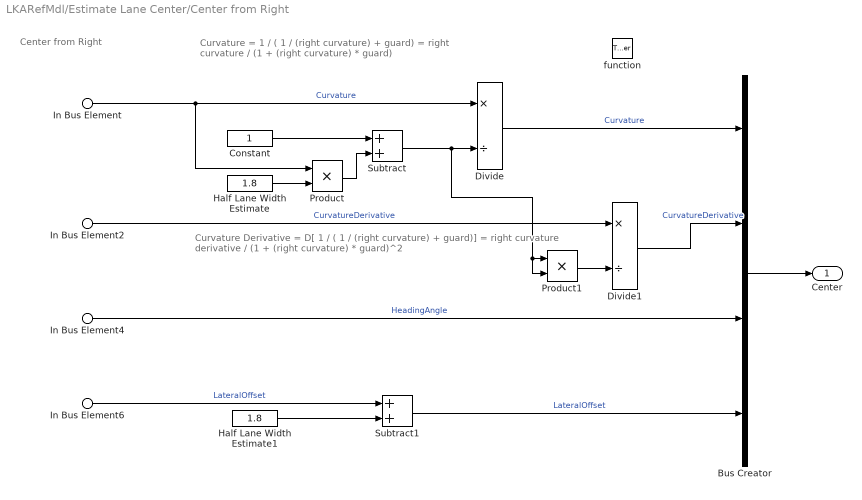
== system LKARefMdl/Estimate Lane Center/Center from Right ==
  note: Center from Right
  note: Curvature
      | = 1 / ( 1 / (right curvature) + guard)
      | = right curvature / (1 + (right curvature) * guard)
  note: Curvature Derivative
      | = D[ 1 / ( 1 / (right curvature) + guard)]
      | = right curvature derivative / (1 + (right curvature) * guard)^2
  In Bus Element : Inport  PortName=Lanes  Element=Right.Curvature
  In Bus Element2 : Inport  PortName=Lanes  Element=Right.CurvatureDerivative
  In Bus Element4 : Inport  PortName=Lanes  Element=Right.HeadingAngle
  In Bus Element6 : Inport  PortName=Lanes  Element=Right.LateralOffset
  function : TriggerPort  TriggerType=function-call  VariantControl=Variant
  Bus Creator : BusCreator  Inputs=4
  Constant : Constant  OutDataTypeStr=Inherit: Inherit via back propagation
  Divide : Product  Inputs=*/
  Divide1 : Product  Inputs=*/
  Half Lane Width Estimate : Constant  Value=1.8  OutDataTypeStr=Inherit: Inherit via back propagation
  Half Lane Width Estimate1 : Constant  Value=1.8  OutDataTypeStr=Inherit: Inherit via back propagation
  Product : Product
  Product1 : Product
  Subtract : Sum
  Subtract1 : Sum
  Center : Outport  VectorParamsAs1DForOutWhenUnconnected=off
  wires:
  In Bus Element2/1 -> Divide1/1  "CurvatureDerivative"
  Divide1/1 -> Bus Creator/2  "CurvatureDerivative"
  Product1/1 -> Divide1/2
  In Bus Element4/1 -> Bus Creator/3  "HeadingAngle"
  Half Lane Width Estimate1/1 -> Subtract1/2
  In Bus Element6/1 -> Subtract1/1  "LateralOffset"
  Divide/1 -> Bus Creator/1  "Curvature"
  Subtract1/1 -> Bus Creator/4  "LateralOffset"
  Bus Creator/1 -> Center/1
  In Bus Element/1 -> Product/1, Divide/1  "Curvature"
  Subtract/1 -> Product1/2, Product1/1, Divide/2
  Constant/1 -> Subtract/1
  Product/1 -> Subtract/2
  Half Lane Width Estimate/1 -> Product/2

== system LKARefMdl/Longitudinal Speed Control/If Action Subsystem2 ==
  In1 : Inport
  Action Port : ActionPort
  Out1 : Outport
  wires:
  In1/1 -> Out1/1

== system LKARefMdl/Longitudinal Speed Control/If Action Subsystem3 ==
  In1 : Inport
  Action Port : ActionPort
  Out1 : Outport
  wires:
  In1/1 -> Out1/1

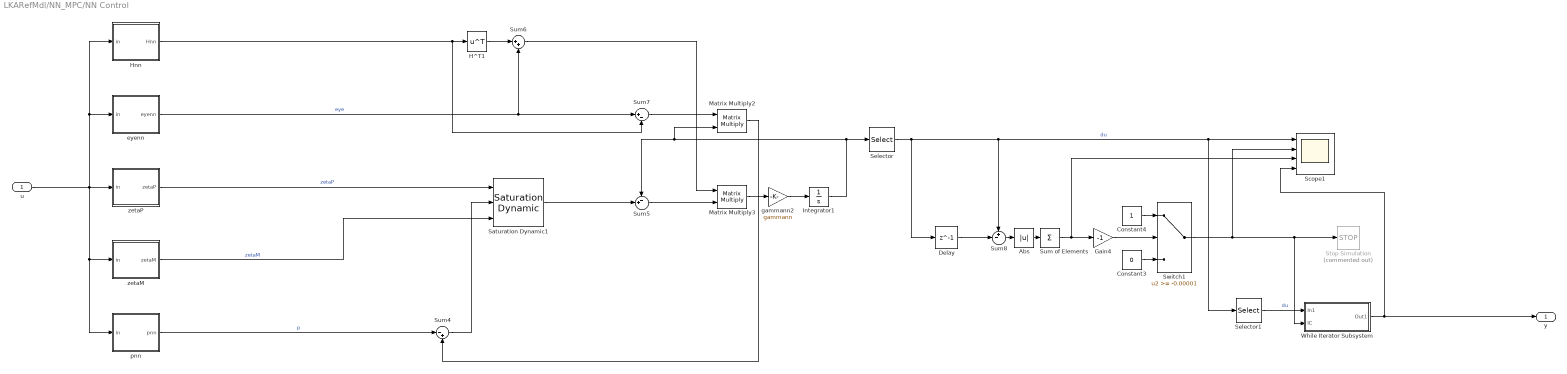
== system LKARefMdl/NN_MPC/NN Control ==
  u : Inport
  Abs : Abs
  Constant3 : Constant  Value=0
  Constant4 : Constant
  Delay : Delay  DelayLength=1  SampleTime=Ts
  Gain4 : Gain  Gain=-1
  H^T1 : Math  Operator=transpose  SaturateOnIntegerOverflow=on
  Hnn : MATLAB Function  TreatAsAtomicUnit=on
  Integrator1 : Integrator  InitialCondition=.10*(rand(numbConstr,1)-0.5)
  Matrix Multiply2 : Product  Multiplication=Matrix(*)
  Matrix Multiply3 : Product  Multiplication=Matrix(*)
  Saturation Dynamic1 : simulink/Discontinuities/Saturation Dynamic  OutMin=[]  OutMax=[]  OutDataTypeStr=Inherit: Same as second input  OutDataType=fixdt(1, 16)  OutScaling=2^-10  DoSatur=off
  Scope1 : Scope  NumInputPorts=4
  Selector : Selector  InputPortWidth=numbConstr  IndexOptions=Index vector (dialog)  Indices=[1:nc]  OutputSizes=1
  Selector1 : Selector  InputPortWidth=nc  IndexOptions=Index vector (dialog)  Indices=[1]  OutputSizes=1
  Stop Simulation : Stop  Commented=on
  Sum of Elements : Sum  Inputs=+
  Sum4 : Sum  Inputs=|-+
  Sum5 : Sum  Inputs=-+|
  Sum6 : Sum  Inputs=|++
  Sum7 : Sum  Inputs=|+-
  Sum8 : Sum  Inputs=+-|
  Switch1 : Switch  Threshold=-0.00001
  While Iterator Subsystem : Subsystem  TreatAsAtomicUnit=on
  eyenn : MATLAB Function  TreatAsAtomicUnit=on
  gammann2 : Gain  Gain=gammann
  pnn : MATLAB Function  TreatAsAtomicUnit=on
  zetaM : MATLAB Function  TreatAsAtomicUnit=on
  zetaP : MATLAB Function  TreatAsAtomicUnit=on
  y : Outport
  wires:
  Selector/1 -> Delay/1, Sum8/1, Selector1/1, Scope1/1  "du"
  Constant3/1 -> Switch1/3
  Switch1/1 -> While Iterator Subsystem/2(IC), Stop Simulation/1, Scope1/2
  Gain4/1 -> Switch1/2
  While Iterator Subsystem/1(Out1) -> y/1, Scope1/4
  Delay/1 -> Sum8/2
  Abs/1 -> Sum of Elements/1
  Sum of Elements/1 -> Gain4/1, Scope1/3
  Constant4/1 -> Switch1/1
  gammann2/1 -> Integrator1/1
  Integrator1/1 -> Matrix Multiply2/2, Sum5/1, Selector/1
  Matrix Multiply3/1 -> gammann2/1
  H^T1/1 -> Sum6/1
  pnn/1(pnn) -> Sum4/1  "p"
  Matrix Multiply2/1 -> Sum4/2
  Sum8/1 -> Abs/1
  Sum4/1 -> Saturation Dynamic1/2
  zetaP/1(zetaP) -> Saturation Dynamic1/1  "zetaP"
  zetaM/1(zetaM) -> Saturation Dynamic1/3  "zetaM"
  Saturation Dynamic1/1 -> Sum5/2
  eyenn/1(eyenn) -> Sum6/2, Sum7/1  "eye"
  Sum5/1 -> Matrix Multiply3/2
  Selector1/1 -> While Iterator Subsystem/1(In1)  "du"
  u/1 -> Hnn/1(in), eyenn/1(in), zetaM/1(in), pnn/1(in), zetaP/1(in)
  Sum7/1 -> Matrix Multiply2/1
  Sum6/1 -> Matrix Multiply3/1
  Hnn/1(Hnn) -> Sum7/2, H^T1/1

== system LKARefMdl/NN_MPC/NN Control/While Iterator Subsystem ==
  In1 : Inport
  IC : Inport  Port=2
  While Iterator : WhileIterator
  Out1 : Outport
  wires:
  IC/1 -> While Iterator/2
  In1/1 -> Out1/1

== matlab function LKARefMdl/NN_MPC/NN Control/zetaM ==
  data: in input; zetaM output size=numbConstr; UU data_store_memory; F data_store_memory; Phi2 data_store_memory; np parameter; gains data_store_memory; Phi1 data_store_memory; v data_store_memory; Ts data_store_memory; nc parameter
function zetaM = zetaM(in, np, nc)

    global F Phi2 gains Phi1 UU
    
   
    bigNumber = 100000;
    singleConstraint = [1 bigNumber*ones(1,nc-1)]';
    
    dumin = -0.1;
    
    xiM = ones(nc,1)*dumin;%.*singleConstraint;
    zetaM = [xiM; bigNumber*zeros(2*nc+2*np,1)]; 
    

end

== matlab function LKARefMdl/Estimate Lane Center/MATLAB Function ==
  data: lanes input
  events: fcnLeftAndRight output FUNCTION_CALL_EVENT; fcnLeftOnly output FUNCTION_CALL_EVENT; fcnRightOnly output FUNCTION_CALL_EVENT; fcnNone output FUNCTION_CALL_EVENT
function fcn(lanes)

leftStrength  = lanes.Left.Strength;
rightStrength = lanes.Right.Strength;

if (leftStrength > 0) && (rightStrength > 0)
   fcnLeftAndRight();
   
elseif leftStrength > 0
    fcnLeftOnly();
    
elseif rightStrength > 0
    fcnRightOnly();
    
else
    fcnNone();
end

== matlab function LKARefMdl/Estimate Lane Center/Preview Curvature ==
  data: rho output; Curvature0 input; dCurvature input; Vx input; Ts parameter; PredictionHorizon parameter
function rho = predictCurvature(Curvature0,dCurvature,Vx, Ts, PredictionHorizon)
% Curvature0 = initial curvature per unit length                  [1/m]
% dCurvature = (constant) derivative of curvature per unit length [1/m^2]
% CurvatureLength = length for which the clothoid model is valid [m]
% Vx = speed of vehicle

% We want to export a set of curvatures at a uniform sample time ahead.
% t is this vector which goes up to 1 second in the future or having
% enough time to reach the known length in curvature (whichever is smaller)

% To enable truncation by curvelength, mark output "rho" as varsize
%t = 0:Ts:min(1,CurvatureLength/Vx);

t = zeros(PredictionHorizon+1,1);
for i=1:numel(t)
    t(i) = (i-1).*Ts;
end

% We compute the curvature vector rho(t) using the specified clothoid model
rho = Curvature0 + dCurvature*Vx*t;

== matlab function LKARefMdl/NN_MPC/NN Control/pnn ==
  data: in input; pnn output size=numbConstr; UU data_store_memory; F data_store_memory; Phi2 data_store_memory; np parameter; gains data_store_memory; Phi1 data_store_memory; v data_store_memory; Ts data_store_memory; nc parameter
function pnn = pnn(in, np, nc)

    global F Phi2 gains Phi1 
    
    % constraints values
    umin = -0.5;
    umax = 0.5;
    ymin = -0.25;
    ymax = 0.25;

    
    curvature = in(1:np);

    % actual speed
    velocity = in(30+2);
    
    if velocity >= 9
        vint = int8(velocity);
    else
        vint = int8(9);
    end
    
    % state
    xk = in(30+3:30+7); % X_k = [x_k u_k]
    psiPrim = curvature.*velocity;
    
    gain = gains(vint-7,:);
    w_x = gain(2:6);
    w_x1 = repmat(w_x,1,np);
    W_x = diag(w_x1);
    
    Phi2n = Phi2(1:length(w_x):end,:);
    Fn = F(1:length(w_x):end,:);
    C1 = ones(nc,1);  
    
    qnn = 2*((F*xk)'*W_x*Phi1 + (Phi2*psiPrim)'*W_x*Phi1)';
    bnn = [-umin*ones(nc,1) + C1*xk(end);...
        umax*ones(nc,1) - C1*xk(end);...
        -ymin*ones(np,1) + Fn*xk + Phi2n*psiPrim;...
        ymax*ones(np,1) - Fn*xk - Phi2n*psiPrim...
        ];
    pnn = [qnn; -bnn]; 

end

== matlab function LKARefMdl/NN_MPC/MATLAB Function1 ==
  data: y output; pp data_store_memory
function y = fcn
%#codegen
global sqrp;
y = sqrp;

== matlab function LKARefMdl/NN_MPC/Bayes // Const Speed ==
  data: in input; u output; UU data_store_memory; F data_store_memory; Phi2 data_store_memory; np data_store_memory; gains data_store_memory; Phi1 data_store_memory; v data_store_memory; Ts data_store_memory; nc data_store_memory
%%%%%%%%%%%%%%%%%%%%%%%%%%%%%%%%%%%%%%%%%%%%%%%%%%%%%%%%%%%%%%%%%%%%%%%%%%%%%%%%%%%%%
% Lateral MPC controller for Bayesian Optimization or constant velocity
% case
% author: Wojciech Stróżecki 2021 
%%%%%%%%%%%%%%%%%%%%%%%%%%%%%%%%%%%%%%%%%%%%%%%%%%%%%%%%%%%%%%%%%%%%%%%%%%%%%%%%%%%%%

function u = MPC_Controls_Bayes(in)

    global F Phi2 np nc gains Phi1 UU
    
    % reference goal speed based on the curvature
    curvature = in(1:np);

    % actual speed
    velocity = in(30+2);
    
    % state
    X_k = in(30+3:30+7); % X_k = [x_k u_k]
    psiPrim = curvature.*velocity;

%     % unconstrained control:
%     Du = UU * (F * X_k + Phi2 * psiPrim);
%     du = double(Du(1,1));
%     fu = du + X_k(end); 

    % constrained control:
    
    % gain contains one set of 6 gains
%     % the case for optimal set:
%     gain = gains(vint-7,:);

    % the case for Bayesian Optimization (UU)
    gain = UU;
    fu = MPC_Constrained_Contro(Phi1,Phi2,F,np,nc,gain,X_k,psiPrim);
    u = [fu; 1];
    
    
end


%%%%%%%%%%%%%%%%%%%%%%%%%%%%%%%%%%%%%%%%%%%%%%%%%%%%%%%%%%%%%%%%%%%%%%%%%%
%%%%%%%%%%%%%%%%%%%%%%%%%%%%%%%%%%%%%%%%%%%%%%%%%%%%%%%%%%%%%%%%%%%%%%%%%%
%%%%%%%%%%%%%%%%%%%%%%%%%%%%%%%%%%%%%%%%%%%%%%%%%%%%%%%%%%%%%%%%%%%%%%%%%%

function u = MPC_Constrained_Contro(Phi1,Phi2,F,np,nc,gains,xk,psiPrim)

    w_x = gains(2:6);
    w_x1 = repmat(w_x,1,np);
    W_x = diag(w_x1);
    w_u = gains(7)*ones(nc,1)';
    W_u = diag(w_u);

    % constraints on x1 only require transformation og F, Phi1 and Phi2 m-x
    Phi1n = Phi1(1:length(w_x):end,:);
    Phi2n = Phi2(1:length(w_x):end,:);
    Fn = F(1:length(w_x):end,:);


    
    
    
    % constraints values
    umin = -0.5;
    umax = 0.5;
    dumin = -0.1;
    dumax = 0.1;
    ymin = -0.35;
    ymax = 0.35;

    % QP variables
    C1 = ones(nc,1);
    C2 = tril(ones(nc,nc));
    Eo = 2*(Phi1'*W_x*Phi1 + W_u);
%     invEo = inv(Eo);
    Fo = 2*((F*xk)'*W_x*Phi1 + (Phi2*psiPrim)'*W_x*Phi1)';
    Mo = [-eye(nc);...
        eye(nc);...
        -C2;...
        C2;...
        -Phi1n;...
        Phi1n...
        ];
    gamma = [-dumin*ones(nc,1);...
        dumax*ones(nc,1);...
        -umin*ones(nc,1) + C1*xk(end);...
        umax*ones(nc,1) - C1*xk(end);...
        -ymin*ones(np,1) + Fn*xk + Phi2n*psiPrim;...
        ymax*ones(np,1) - Fn*xk - Phi2n*psiPrim...
        ];
    
    % Iterative constraint violation check
%     lambda = -inv(Mo*invEo*Mo')*(gamma + Mo*invEo*Fo');
%     find(lambda >= 0)





% Solving QP with Active set - will break for more than nc active constraints:
% %     if all(lambda < 0)
%     if det(Mo*(Eo\Mo')) <= 0
%         Du = -invEo*Fo';
%         du = Du(1,1);
%         u = du + xk(end);
%     else
%         lambda = -inv(Mo*invEo*Mo')*(gamma + Mo*invEo*Fo');
%         while ~all(lambda >= 0)
%             act = find(lambda >= 0);
%             gammaact = gamma(act,:);
%             Moact = Mo(act,:);
%             lambda = -inv(Moact*invEo*Moact')*(gammaact + Moact*invEo*Fo');
%         end
%         Du = -invEo*(Fo + Moact*lambda);
%         du = Du(1,1);
%         u = du + xk(end); 
%     end

% Solving QP with Hildreth
    Du = BookHildret(Eo,Fo,Mo,gamma);
    du = Du(1,1);
    u = du + xk(end);
% Important program features
    fi_ut = 14.5;
end





%%%%%%%%%%%%%%%%%%%%%%%%%%%%%%%%%%%%%%%%%%%%%%%%%%%%%%%%%%%%%%%%%%%%%%%%%%
%%%%%%%%%%%%%%%%%%%%%%%%%%%%%%%%%%%%%%%%%%%%%%%%%%%%%%%%%%%%%%%%%%%%%%%%%%
%%%%%%%%%%%%%%%%%%%%%%%%%%%%%%%%%%%%%%%%%%%%%%%%%%%%%%%%%%%%%%%%%%%%%%%%%%


function eta = BookHildret(H,f,A_cons,b)

%     E=H;
%     F=f;
%     M=A_cons;
%     gamma=b;
%     eta =x;
    [n1,m1]=size(A_cons);
    eta=-H\f;
    kk=0;

    for i=1:n1
        if  (A_cons(i,:)*eta>b(i))
            kk=kk+1;
        else
            kk=kk+0;
        end
    end
    
    if (kk==0)
        return;
    end
        
   
    P=A_cons*(H\A_cons');
    d=(A_cons*(H\f)+b);
    [n,m]=size(d);
    x_ini=zeros(n,m);
    lambda=x_ini;
    al=10;

    for km=1:100
    
        %find the elements in the solution vector one by one
        % km could be larger if the Lagranger multiplier has a slow
        % convergence rate.
        lambda_p=lambda;

        for i=1:n
            w= P(i,:)*lambda-P(i,i)*lambda(i,1);
            w=w+d(i,1);
            la=-w/P(i,i);
            lambda(i,1)=max(0,la);
        end
        
        al=(lambda-lambda_p)'*(lambda-lambda_p);
        if (al<10e-8)
            break;
        end
    end
    eta=-H\f -H\A_cons'*lambda;
end
